simulink subsystem "TV_2WD_NO_REGEN"  (R2023b)
settings: Solver=VariableStepAuto  StartTime=0.0  StopTime=10.0  RelTol=1e-3
settings Model: Creator=Inver  LastModifiedBy=Inver

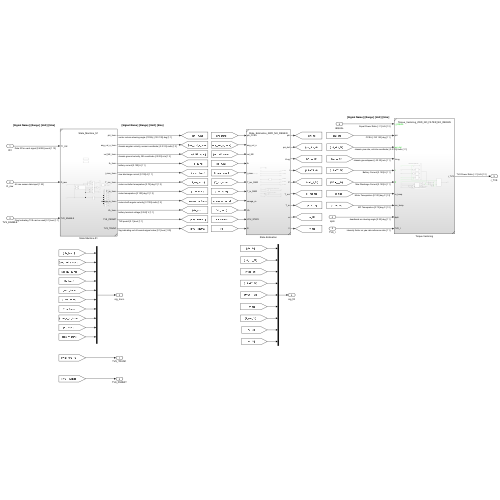
[thumbnail: Simulink's stored preview of the top-level diagram]
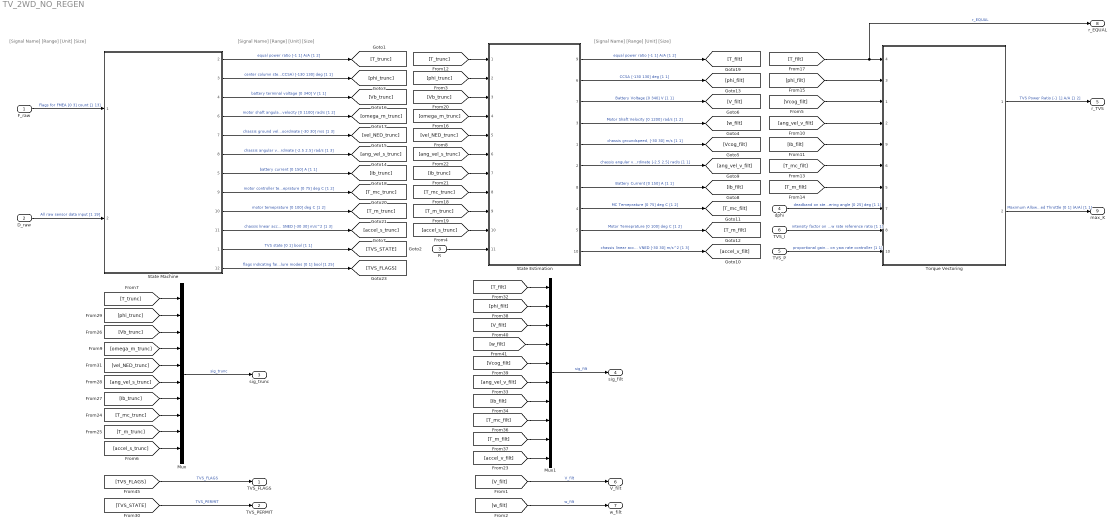
== system TV_2WD_NO_REGEN ==
  note: [Signal Name] [Range] [Unit] [Size]
  note: [Signal Name] [Range] [Unit] [Size]
  note: [Signal Name] [Range] [Unit] [Size]
  F_raw : Inport
  D_raw : Inport  Port=2
  R : Inport  Port=3
  dphi : Inport  Port=4
  TVS_P : Inport  Port=5
  TVS_I : Inport  Port=6
  Mux : Mux  Inputs=10
  Mux1 : Mux  Inputs=10
  State Estimation : Subsystem  ReferencedSubsystem=State_Estimation_2WD_NO_REGEN
      settings: PortSchema="{\"entries\":[{\"content\":{\"sides\":[{\"content\":{\"connectorIds\":[\"In1\",\"In2\",\"In3\",\"In4\",\"In5\",\"In6\",\"In7\",\"In8\",\"In9\",\"In10\",\"In11\"]},\"type\":\"ConnectorPlacement.EquallySpacedRectSide\",\"uuid\":\"a788c4af-c868-4742-81ae-137d8550b7dd\"},{\"content\":{\"connectorIds\":[\"Out9\",\"Out6\",\"Out7\",\"Out3\",\"Out1\",\"Out2\",\"Out8\",\"Out4\",\"Out5\",\"Out10\"],\"side\":\"RIGHT\"},\"type\":\"ConnectorPlacement.EquallySpacedRectSide\",\"uuid\":\"40c1d3ed-7f96-4f50-8201-1fa73cbd293c\"},{\"content\":{\"side\":\"TOP\"},\"type\":\"ConnectorPlacement.EquallySpacedRectSide\",\"uuid\":\"412486a9-9897-40de-926c-efa6067c47b5\"}]},\"type\":\"ConnectorPlacement.EquallySpacedConnector\",\"uuid\":\"e2349428-ea4b-4d6c-9a0f-70e14711b204\"}],\"packageUris\":[\"http://schema.mathworks.com/mf0/Connector/R2020b\"],\"version\":\"1.0\"}"
  State Machine : Subsystem  ReferencedSubsystem=State_Machine_S1
      settings: PortSchema="{\"entries\":[{\"content\":{\"sides\":[{\"content\":{\"connectorIds\":[\"In1\",\"In2\"]},\"type\":\"ConnectorPlacement.EquallySpacedRectSide\",\"uuid\":\"3ad5cc8f-5c24-495b-b7bf-c12b21ca6743\"},{\"content\":{\"connectorIds\":[\"Out2\",\"Out3\",\"Out4\",\"Out6\",\"Out7\",\"Out8\",\"Out5\",\"Out9\",\"Out10\",\"Out11\",\"Out1\",\"Out12\"],\"side\":\"RIGHT\"},\"type\":\"ConnectorPlacement.EquallySpacedRectSide\",\"uuid\":\"199951c7-79be-4b7a-80a1-2c2fec8c516f\"},{\"content\":{\"side\":\"TOP\"},\"type\":\"ConnectorPlacement.EquallySpacedRectSide\",\"uuid\":\"296cd14f-6cd9-481e-92b9-c36b65280b3a\"}]},\"type\":\"ConnectorPlacement.EquallySpacedConnector\",\"uuid\":\"592bd7cc-8272-4bf2-9b34-0f5ee02d28bc\"}],\"packageUris\":[\"http://schema.mathworks.com/mf0/Connector/R2020b\"],\"version\":\"1.0\"}"
  Torque Vectoring : Subsystem  ReferencedSubsystem=Torque_Vectoring_2WD_NO_FILTER_NO_REGEN
      settings: PortSchema="{\"entries\":[{\"content\":{\"sides\":[{\"content\":{\"connectorIds\":[\"In4\",\"In3\",\"In1\",\"In2\",\"In9\",\"In6\",\"In5\",\"In7\",\"In8\",\"In10\"]},\"type\":\"ConnectorPlacement.EquallySpacedRectSide\",\"uuid\":\"e5337710-7afc-44d5-961b-efcd80b22325\"},{\"content\":{\"connectorIds\":[\"Out1\",\"Out2\"],\"side\":\"RIGHT\"},\"type\":\"ConnectorPlacement.EquallySpacedRectSide\",\"uuid\":\"7e97e5bc-3983-40c2-bdf4-f229f862f80b\"},{\"content\":{\"side\":\"TOP\"},\"type\":\"ConnectorPlacement.EquallySpacedRectSide\",\"uuid\":\"1eebe57d-188b-4569-998a-307371d30e4f\"}]},\"type\":\"ConnectorPlacement.EquallySpacedConnector\",\"uuid\":\"25a81eaa-afe2-4445-a3db-4a69d15d4e62\"}],\"packageUris\":[\"http://schema.mathworks.com/mf0/Connector/R2020b\"],\"version\":\"1.0\"}"
  TVS_FLAGS : Outport
  TVS_PERMIT : Outport  Port=2
  sig_trunc : Outport  Port=3
  sig_filt : Outport  Port=4
  r_TVS : Outport  Port=5
  V_filt : Outport  Port=6
  w_filt : Outport  Port=7
  r_EQUAL : Outport  Port=8
  max_K : Outport  Port=9
  wires:
  TVS_P/1 -> Torque Vectoring/10  "proportional gain on yaw rate controller [1 1]"
  [accel_v_filt] -> Mux1/10
  [T_m_filt] -> Mux1/9
  [T_mc_filt] -> Mux1/8
  [Ib_filt] -> Mux1/7
  [ang_vel_v_filt] -> Mux1/6
  [Vcog_filt] -> Mux1/5
  [w_filt] -> Mux1/4
  [V_filt] -> Mux1/3
  [phi_filt] -> Mux1/2
  [T_filt] -> Mux1/1
  State Estimation/9 -> [T_filt]  "equal power ratio [-1 1] A/A [1 2]"
  [vel_NED_trunc] -> Mux/5
  [T_trunc] -> Mux/1
  State Estimation/10 -> [accel_v_filt]  "chassis linear acceleration VNED [-30 30] m/s^2 [1 3]"
  [T_trunc] -> State Estimation/1
  [accel_s_trunc] -> State Estimation/10
  State Machine/11 -> [accel_s_trunc]  "chassis linear acceleration SNED [-30 30] m/s^2 [1 3]"
  State Machine/2 -> [T_trunc]  "equal power ratio [-1 1] A/A [1 2]"
  [w_filt] -> w_filt/1  "w_filt"
  [V_filt] -> V_filt/1  "V_filt"
  [T_filt] -> Torque Vectoring/4, r_EQUAL/1  "r_EQUAL"
  TVS_I/1 -> Torque Vectoring/8  "intensity factor on yaw rate reference ratio [1 1]"
  State Machine/3 -> [phi_trunc]  "center column steering angle (CCSA) [-130 130] deg [1 1]"
  [phi_filt] -> Torque Vectoring/3
  [vel_NED_trunc] -> State Estimation/5
  [omega_m_trunc] -> State Estimation/4
  F_raw/1 -> State Machine/1  "Flags for FMEA [0 3] count [1 13]"
  [ang_vel_s_trunc] -> State Estimation/6
  State Estimation/1 -> [Vcog_filt]  "chassis groundspeed, [-30 30] m/s [1 1]"
  State Machine/6 -> [omega_m_trunc]  "motor shaft angular velocity [0 1100] rad/s [1 2]"
  D_raw/1 -> State Machine/2  "All raw sensor data input [1 19]"
  [Vb_trunc] -> Mux/3
  State Estimation/5 -> [T_m_filt]  "Motor Temeprature [0 100] deg C [1 2]"
  [Vb_trunc] -> State Estimation/3
  [ang_vel_s_trunc] -> Mux/6
  [ang_vel_v_filt] -> Torque Vectoring/2
  State Machine/1 -> [TVS_STATE]  "TVS state [0 1] bool [1 1]"
  State Machine/10 -> [T_m_trunc]  "motor temeprature [0 100] deg C [1 2]"
  [T_m_filt] -> Torque Vectoring/5
  State Machine/7 -> [vel_NED_trunc]  "chassis ground velocity, NED coordinate [-30 30] m/s [1 3]"
  [accel_s_trunc] -> Mux/10
  R/1 -> State Estimation/11
  [phi_trunc] -> State Estimation/2
  [omega_m_trunc] -> Mux/4
  [Ib_filt] -> Torque Vectoring/9
  [TVS_STATE] -> TVS_PERMIT/1  "TVS_PERMIT"
  State Estimation/6 -> [phi_filt]  "CCSA [-130 130] deg [1 1]"
  State Machine/9 -> [T_mc_trunc]  "motor controller temeprature [0 75] deg C [1 2]"
  [Ib_trunc] -> Mux/7
  [Ib_trunc] -> State Estimation/7
  [T_mc_trunc] -> Mux/8
  State Machine/5 -> [Ib_trunc]  "battery current [0 150] A [1 1]"
  [Vcog_filt] -> Torque Vectoring/1
  State Machine/4 -> [Vb_trunc]  "battery terminal voltage [0 340] V [1 1]"
  State Estimation/8 -> [Ib_filt]  "Battery Current [0 150] A [1 1]"
  [T_mc_filt] -> Torque Vectoring/6
  [T_m_trunc] -> Mux/9
  State Estimation/2 -> [ang_vel_v_filt]  "chassis angular velocity, vehicle coordinate [-2.5 2.5] rad/s [1 1]"
  State Estimation/7 -> [V_filt]  "Battery Voltage [0 340] V [1 1]"
  [phi_trunc] -> Mux/2
  State Estimation/3 -> [w_filt]  "Motor Shaft Velocity [0 1200] rad/s [1 2]"
  [T_m_trunc] -> State Estimation/9
  Mux1/1 -> sig_filt/1  "sig_filt"
  Mux/1 -> sig_trunc/1  "sig_trunc"
  [T_mc_trunc] -> State Estimation/8
  State Estimation/4 -> [T_mc_filt]  "MC Temeprature [0 75] deg C [1 2]"
  Torque Vectoring/1 -> r_TVS/1  "TVS Power Ratio [-1 1] A/A [1 2]"
  [TVS_FLAGS] -> TVS_FLAGS/1  "TVS_FLAGS"
  State Machine/8 -> [ang_vel_s_trunc]  "chassis angular velocity, sensor coordinate [-2.5 2.5] rad/s [1 3]"
  dphi/1 -> Torque Vectoring/7  "deadband on steering angle [0 25] deg [1 1]"
  State Machine/12 -> [TVS_FLAGS]  "flags indicating failure modes [0 1] bool [1 25]"
  Torque Vectoring/2 -> max_K/1  "Maximum Allowed Throttle [0 1] (A/A) [1 1]"
